simulink model "Model"  (R2024b)
settings: Solver=ode45  StartTime=0.0  StopTime=20  RelTol=1e-3
InitFcn:
  | Design
values from neighbouring files (symbols this model uses):
  A = [0, 1; 0, -1/Tm]    [Design.m]
  B = [0; Km/Tm/gbox.N]    [Design.m]
  C = [1, 0]    [Design.m]
  D = 0    [Design.m]
  K = K(2:end)    [Design.m]
  Ki = K(1)    [Design.m]
  Nr = Nu + K * Nx    [Design.m]
  Nu = tmp(end)    [Design.m]
  Nx = tmp(1:N, 1)    [Design.m]
  Ref = 70    [Design.m]
undefined symbols (not defined in the file or in its folder): daq, drv, ElecDyn, gbox, MechDyn, mot, rads2rpm, RD, sens, Tau_sf, Ts
libraries: simulink_extras x5
settings Model: Creator=Banaan  LastModifiedBy=Banaan

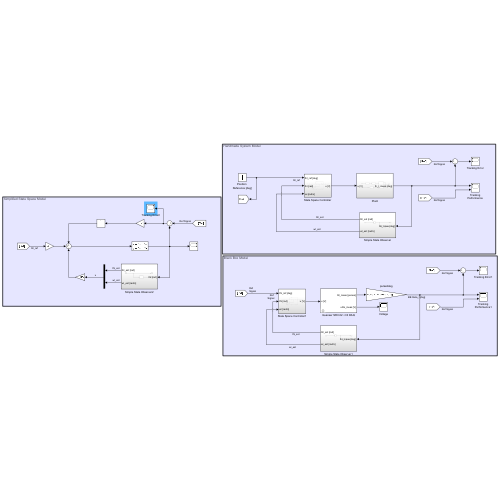
[thumbnail: Simulink's stored preview of the top-level diagram]
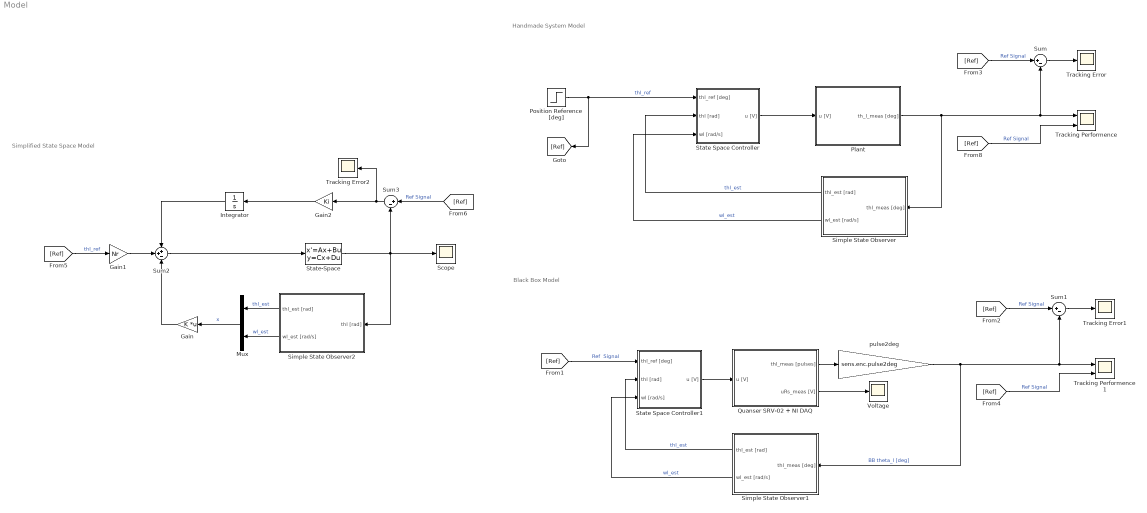
== system Model ==
  note: Simplified State Space Model
  note: Handmade System Model
  note: Black Box Model
  Gain : Gain  Gain=K  Multiplication=Matrix(K*u)
  Gain1 : Gain  Gain=Nr
  Gain2 : Gain  Gain=Ki
  Integrator : Integrator
  Mux : Mux  Inputs=2
  Plant : Subsystem
  Position Reference [deg] : Step  After=Ref  SampleTime=0
  Quanser SRV-02 + NI DAQ : Subsystem  mask(Quanser SRV-02 (with inertial load) + NI DAQ){Ts=0.001, fricType=Coulomb + viscous}
      mask prompts: Ts "NI DAQ Sample Time:"; fricType "Friction model"
      mask help: Quanser SRV-02 (with inertial load) + NI DAQ model.
      mask init:
      | %%  Sensors data
      | 
      | %   shunt resistor
      | sens.curr.Rs = 0.5;                         %   resistance [Ohm]   
      | sens.curr.uRs_std = 0.01;                   %   voltage noise standard dev [V]                           
      | sens.curr.uRs_var = sens.curr.uRs_std^2;	%   voltage noise variance [V^2]
      | 
      | %   Hewlett-Packard HEDS-5540#A06 optical encoder
      | sens.enc.ppr = 500*4;                       %   pulses per rotation
      | sens.enc.pulse2deg = 360/sens.enc.ppr;      %   [pulses] -> [deg]
      | sens.enc.pulse2rad = 2*pi/sens.enc.ppr;     %   [pulses] -> [rad]
      | sens.enc.deg2pulse = sens.enc.ppr/360;      %   [deg] -> [pulses]
      | sens.enc.rad2pulse = sens.enc.ppr/2/pi;     %   [rad] -> [pulses]
      | 
      | 
      | %%  Data acquisition board (daq) data
      | 
      | %   NI PCI-6221 DAC data
      | daq.dac.bits = 16;                                  %   resolution (bits)
      | daq.dac.fs   = 10;                                  %   full scale 
      | daq.dac.q    = 2*daq.dac.fs/(2^daq.dac.bits-1);     %	quantization
      | 
      | %   NI PCI-6221 ADC data
      | daq.adc.bits = 16;                                  %   resolution (bits)
      | daq.adc.fs   = 10;                                  %   full scale (as set in SLDRT Analog Input block)
      | daq.adc.q    = 2*daq.adc.fs/(2^daq.adc.bits-1);     %   quantization
      mask Help:
      | Riccardo Antonello (antonello@dei.unipd.it)
      | 
      | April 24, 2020
      | 
      | Dept. of Information Engineering, University of Padova
      mask TypeOptions fricType: Coulomb + viscous | Karnopp
  Scope : Scope
  Simple State Observer : Subsystem
  Simple State Observer1 : Subsystem
  Simple State Observer2 : Subsystem
  State Space Controller : Subsystem
  State Space Controller1 : Subsystem
  State-Space : StateSpace  A=A  B=B  C=C  D=D  InitialCondition=0
  Sum : Sum  Inputs=|+-
  Sum1 : Sum  Inputs=|+-
  Sum2 : Sum  Inputs=++-
  Sum3 : Sum  Inputs=|+-
  Tracking Performence : Scope  NumInputPorts=2
  Tracking Performence1 : Scope  NumInputPorts=2
  Tracking Error : Scope
  Tracking Error1 : Scope
  Tracking Error2 : Scope
  Voltage : Scope
  pulse2deg : Gain  Gain=sens.enc.pulse2deg
  wires:
  Plant/1(th_l_meas [deg]) -> Sum/2, Tracking Performence/1, Simple State Observer/1(thl_meas [deg])
  Position Reference [deg]/1 -> [Ref], State Space Controller/1(thl_ref [deg])  "thl_ref"
  Quanser SRV-02 + NI DAQ/1(thl_meas [pulses]) -> pulse2deg/1
  pulse2deg/1 -> Simple State Observer1/1(thl_meas [deg]), Tracking Performence1/1, Sum1/2  "BB theta_l [deg]"
  Quanser SRV-02 + NI DAQ/2(uRs_meas [V]) -> Voltage/1
  [Ref] -> State Space Controller1/1(thl_ref [deg])  "Ref  Signal"
  [Ref] -> Tracking Performence/2  "Ref Signal"
  State Space Controller/1(u [V]) -> Plant/1(u [V])
  Simple State Observer/1(thl_est [rad]) -> State Space Controller/2(thl [rad])  "thl_est"
  Simple State Observer/2(wl_est [rad/s]) -> State Space Controller/3(wl [rad/s])  "wl_est"
  [Ref] -> Sum/1  "Ref Signal"
  Sum/1 -> Tracking Error/1
  Sum1/1 -> Tracking Error1/1
  [Ref] -> Sum1/1  "Ref Signal"
  [Ref] -> Tracking Performence1/2  "Ref Signal"
  Simple State Observer1/2(wl_est [rad/s]) -> State Space Controller1/3(wl [rad/s])  "wl_est"
  Simple State Observer1/1(thl_est [rad]) -> State Space Controller1/2(thl [rad])  "thl_est"
  State Space Controller1/1(u [V]) -> Quanser SRV-02 + NI DAQ/1(u [V])
  Simple State Observer2/2(wl_est [rad/s]) -> Mux/2  "wl_est"
  Simple State Observer2/1(thl_est [rad]) -> Mux/1  "thl_est"
  Mux/1 -> Gain/1  "x"
  Gain/1 -> Sum2/3
  Sum2/1 -> State-Space/1
  Gain1/1 -> Sum2/2
  [Ref] -> Gain1/1  "thl_ref"
  [Ref] -> Sum3/1  "Ref Signal"
  Sum3/1 -> Gain2/1, Tracking Error2/1
  State-Space/1 -> Sum3/2, Scope/1, Simple State Observer2/1(thl [rad])
  Gain2/1 -> Integrator/1
  Integrator/1 -> Sum2/1

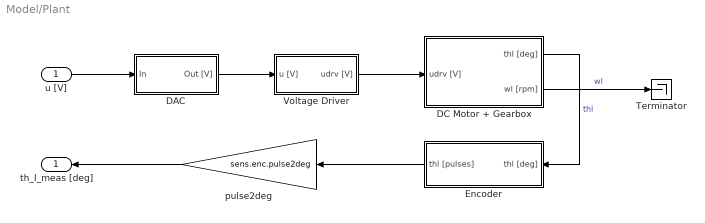
== system Model/Plant ==
  u [V] : Inport
  DAC : Subsystem
  DC Motor + Gearbox : Subsystem
  Encoder : Subsystem
  Terminator : Terminator
  Voltage Driver : Subsystem
  pulse2deg : Gain  Gain=sens.enc.pulse2deg
  th_l_meas [deg] : Outport
  wires:
  DAC/1(Out [V]) -> Voltage Driver/1(u [V])
  Encoder/1(thl [pulses]) -> pulse2deg/1
  u [V]/1 -> DAC/1(In)
  Voltage Driver/1(udrv [V]) -> DC Motor + Gearbox/1(udrv [V])
  DC Motor + Gearbox/2(wl [rpm]) -> Terminator/1  "wl"
  DC Motor + Gearbox/1(thl [deg]) -> Encoder/1(thl [deg])  "thl"
  pulse2deg/1 -> th_l_meas [deg]/1

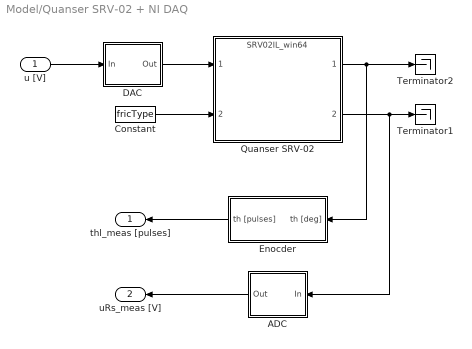
== system Model/Quanser SRV-02 + NI DAQ ==
  u [V] : Inport
  ADC : Subsystem
  Constant : Constant  Value=fricType
  DAC : Subsystem
  Enocder : Subsystem
  Quanser SRV-02 : ModelReference  ModelNameDialog=SRV02IL_win64.slxp  ModelReferenceVersion=1.44  CopyOfModelProtected=on
  Terminator1 : Terminator
  Terminator2 : Terminator
  thl_meas [pulses] : Outport
  uRs_meas [V] : Outport  Port=2
  wires:
  Enocder/1(th [pulses]) -> thl_meas [pulses]/1
  ADC/1(Out) -> uRs_meas [V]/1
  DAC/1(Out) -> Quanser SRV-02/1
  Quanser SRV-02/2 -> ADC/1(In), Terminator1/1
  u [V]/1 -> DAC/1(In)
  Quanser SRV-02/1 -> Enocder/1(th [deg]), Terminator2/1
  Constant/1 -> Quanser SRV-02/2

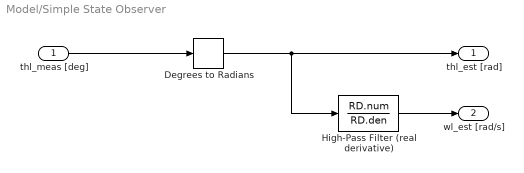
== system Model/Simple State Observer ==
  thl_meas [deg] : Inport
  Degrees to Radians : simulink_extras/Transformations/Degrees to Radians
  High-Pass Filter (real derivative) : TransferFcn  Numerator=RD.num  Denominator=RD.den
  thl_est [rad] : Outport
  wl_est [rad/s] : Outport  Port=2
  wires:
  thl_meas [deg]/1 -> Degrees to Radians/1
  High-Pass Filter (real derivative)/1 -> wl_est [rad/s]/1
  Degrees to Radians/1 -> High-Pass Filter (real derivative)/1, thl_est [rad]/1

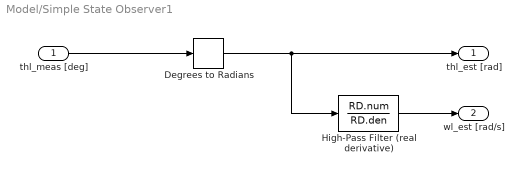
== system Model/Simple State Observer1 ==
  thl_meas [deg] : Inport
  Degrees to Radians : simulink_extras/Transformations/Degrees to Radians
  High-Pass Filter (real derivative) : TransferFcn  Numerator=RD.num  Denominator=RD.den
  thl_est [rad] : Outport
  wl_est [rad/s] : Outport  Port=2
  wires:
  High-Pass Filter (real derivative)/1 -> wl_est [rad/s]/1
  Degrees to Radians/1 -> High-Pass Filter (real derivative)/1, thl_est [rad]/1
  thl_meas [deg]/1 -> Degrees to Radians/1

== system Model/Simple State Observer2 ==
  thl [rad] : Inport
  High-Pass Filter (real derivative) : TransferFcn  Numerator=RD.num  Denominator=RD.den
  thl_est [rad] : Outport
  wl_est [rad/s] : Outport  Port=2
  wires:
  High-Pass Filter (real derivative)/1 -> wl_est [rad/s]/1
  thl [rad]/1 -> thl_est [rad]/1, High-Pass Filter (real derivative)/1

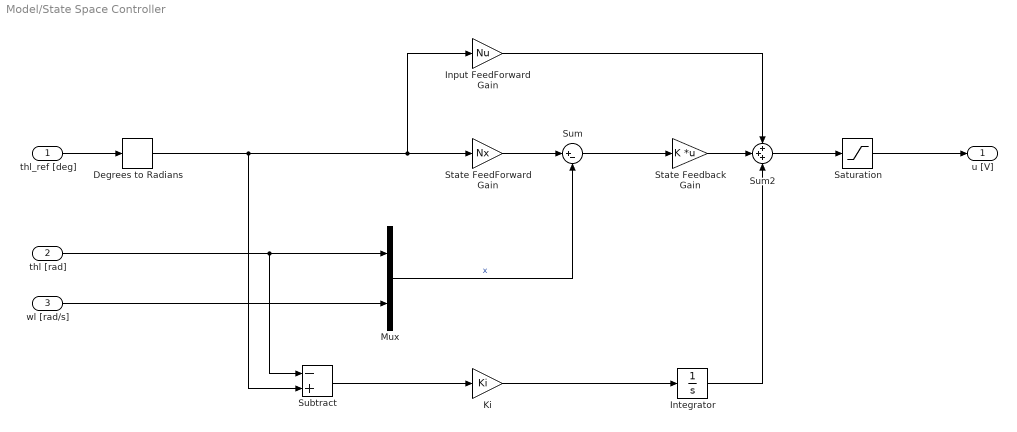
== system Model/State Space Controller ==
  thl_ref [deg] : Inport
  thl [rad] : Inport  Port=2
  wl [rad/s] : Inport  Port=3
  Degrees to Radians : simulink_extras/Transformations/Degrees to Radians
  Input FeedForward Gain : Gain  Gain=Nu
  Integrator : Integrator
  Ki : Gain  Gain=Ki
  Mux : Mux  Inputs=2
  Saturation : Saturate  UpperLimit=daq.adc.fs  LowerLimit=-daq.adc.fs
  State FeedForward Gain : Gain  Gain=Nx
  State Feedback Gain : Gain  Gain=K  Multiplication=Matrix(K*u)
  Subtract : Sum  Inputs=-+
  Sum : Sum  Inputs=|+-
  Sum2 : Sum  Inputs=+++
  u [V] : Outport
  wires:
  Sum/1 -> State Feedback Gain/1
  Mux/1 -> Sum/2  "x"
  thl_ref [deg]/1 -> Degrees to Radians/1
  State FeedForward Gain/1 -> Sum/1
  State Feedback Gain/1 -> Sum2/2
  Input FeedForward Gain/1 -> Sum2/1
  Sum2/1 -> Saturation/1
  Saturation/1 -> u [V]/1
  Degrees to Radians/1 -> Subtract/2, Input FeedForward Gain/1, State FeedForward Gain/1
  thl [rad]/1 -> Subtract/1, Mux/1
  wl [rad/s]/1 -> Mux/2
  Subtract/1 -> Ki/1
  Ki/1 -> Integrator/1
  Integrator/1 -> Sum2/3

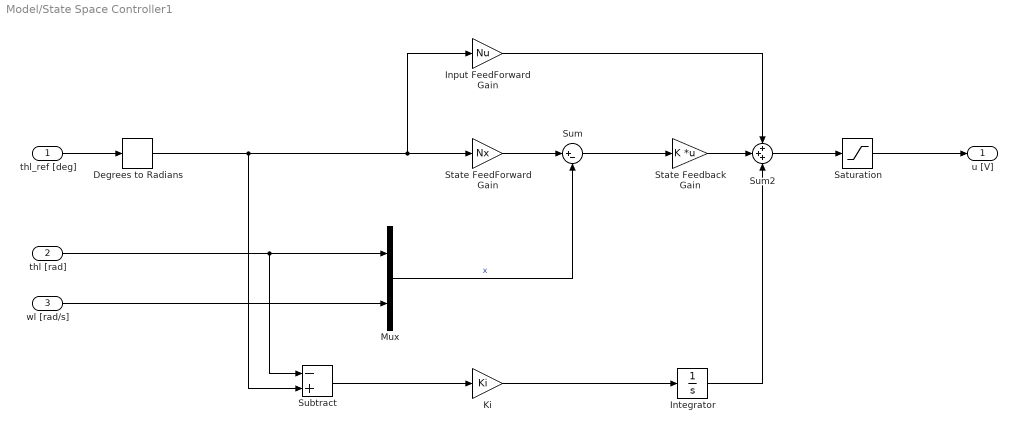
== system Model/State Space Controller1 ==
  thl_ref [deg] : Inport
  thl [rad] : Inport  Port=2
  wl [rad/s] : Inport  Port=3
  Degrees to Radians : simulink_extras/Transformations/Degrees to Radians
  Input FeedForward Gain : Gain  Gain=Nu
  Integrator : Integrator
  Ki : Gain  Gain=Ki
  Mux : Mux  Inputs=2
  Saturation : Saturate  UpperLimit=daq.adc.fs  LowerLimit=-daq.adc.fs
  State FeedForward Gain : Gain  Gain=Nx
  State Feedback Gain : Gain  Gain=K  Multiplication=Matrix(K*u)
  Subtract : Sum  Inputs=-+
  Sum : Sum  Inputs=|+-
  Sum2 : Sum  Inputs=+++
  u [V] : Outport
  wires:
  Saturation/1 -> u [V]/1
  Sum/1 -> State Feedback Gain/1
  wl [rad/s]/1 -> Mux/2
  Ki/1 -> Integrator/1
  Subtract/1 -> Ki/1
  State FeedForward Gain/1 -> Sum/1
  Sum2/1 -> Saturation/1
  thl_ref [deg]/1 -> Degrees to Radians/1
  Degrees to Radians/1 -> Subtract/2, Input FeedForward Gain/1, State FeedForward Gain/1
  thl [rad]/1 -> Subtract/1, Mux/1
  Input FeedForward Gain/1 -> Sum2/1
  Mux/1 -> Sum/2  "x"
  State Feedback Gain/1 -> Sum2/2
  Integrator/1 -> Sum2/3

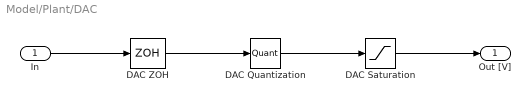
== system Model/Plant/DAC ==
  In : Inport
  DAC Quantization : Quantizer  QuantizationInterval=daq.dac.q
  DAC Saturation : Saturate  UpperLimit=daq.dac.fs  LowerLimit=-daq.dac.fs
  DAC ZOH : ZeroOrderHold  SampleTime=Ts
  Out [V] : Outport
  wires:
  DAC Quantization/1 -> DAC Saturation/1
  DAC ZOH/1 -> DAC Quantization/1
  DAC Saturation/1 -> Out [V]/1
  In/1 -> DAC ZOH/1

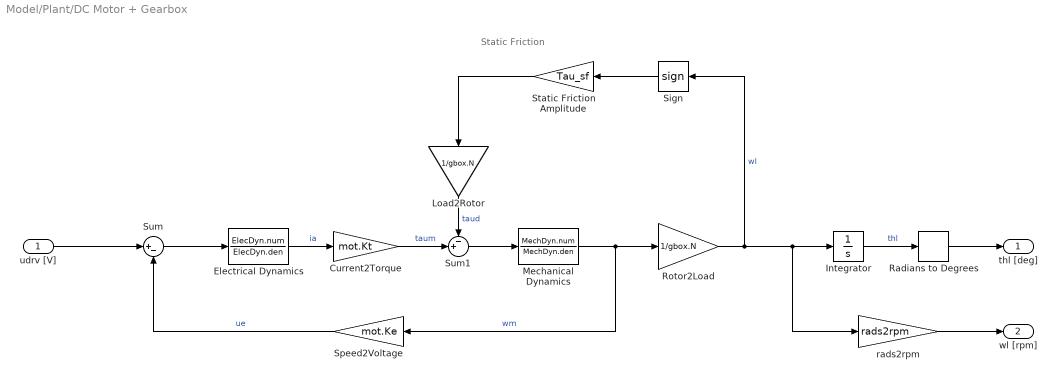
== system Model/Plant/DC Motor + Gearbox ==
  note: Static Friction
  udrv [V] : Inport
  Current2Torque : Gain  Gain=mot.Kt
  Electrical Dynamics : TransferFcn  Numerator=ElecDyn.num  Denominator=ElecDyn.den
  Integrator : Integrator
  Load2Rotor : Gain  Gain=1/gbox.N
  Mechanical Dynamics : TransferFcn  Numerator=MechDyn.num  Denominator=MechDyn.den
  Radians to Degrees : simulink_extras/Transformations/Radians to Degrees
  Rotor2Load : Gain  Gain=1/gbox.N
  Sign : Signum  ZeroCross=off
  Speed2Voltage : Gain  Gain=mot.Ke
  Static Friction Amplitude : Gain  Gain=Tau_sf
  Sum : Sum  Inputs=|+-
  Sum1 : Sum  Inputs=-+|
  rads2rpm : Gain  Gain=rads2rpm
  thl [deg] : Outport
  wl [rpm] : Outport  Port=2
  wires:
  Rotor2Load/1 -> rads2rpm/1, Integrator/1, Sign/1  "wl"
  Electrical Dynamics/1 -> Current2Torque/1  "ia"
  Sum1/1 -> Mechanical Dynamics/1
  Speed2Voltage/1 -> Sum/2  "ue"
  Load2Rotor/1 -> Sum1/1  "taud"
  Radians to Degrees/1 -> thl [deg]/1
  Mechanical Dynamics/1 -> Speed2Voltage/1, Rotor2Load/1  "wm"
  Sum/1 -> Electrical Dynamics/1
  Integrator/1 -> Radians to Degrees/1  "thl"
  Current2Torque/1 -> Sum1/2  "taum"
  rads2rpm/1 -> wl [rpm]/1
  Sign/1 -> Static Friction Amplitude/1
  Static Friction Amplitude/1 -> Load2Rotor/1
  udrv [V]/1 -> Sum/1

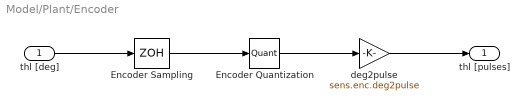
== system Model/Plant/Encoder ==
  thl [deg] : Inport
  Encoder Quantization : Quantizer  QuantizationInterval=daq.adc.q
  Encoder Sampling : ZeroOrderHold  SampleTime=Ts
  deg2pulse : Gain  Gain=sens.enc.deg2pulse
  thl [pulses] : Outport
  wires:
  Encoder Sampling/1 -> Encoder Quantization/1
  Encoder Quantization/1 -> deg2pulse/1
  thl [deg]/1 -> Encoder Sampling/1
  deg2pulse/1 -> thl [pulses]/1

== system Model/Plant/Voltage Driver ==
  u [V] : Inport
  Driver Dynamics : TransferFcn  Numerator=drv.dcgain  Denominator=[drv.Tc, 1]
  Driver Saturation : Saturate  UpperLimit=drv.outmax  LowerLimit=-drv.outmax
  udrv [V] : Outport
  wires:
  Driver Dynamics/1 -> Driver Saturation/1
  u [V]/1 -> Driver Dynamics/1
  Driver Saturation/1 -> udrv [V]/1

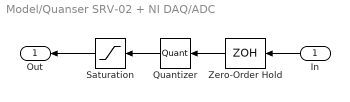
== system Model/Quanser SRV-02 + NI DAQ/ADC ==
  In : Inport
  Quantizer : Quantizer  QuantizationInterval=daq.adc.q
  Saturation : Saturate  UpperLimit=daq.adc.fs  LowerLimit=-daq.adc.fs
  Zero-Order Hold : ZeroOrderHold  SampleTime=Ts
  Out : Outport
  wires:
  Saturation/1 -> Out/1
  In/1 -> Zero-Order Hold/1
  Quantizer/1 -> Saturation/1
  Zero-Order Hold/1 -> Quantizer/1

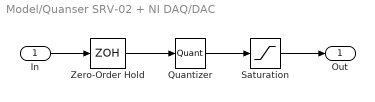
== system Model/Quanser SRV-02 + NI DAQ/DAC ==
  In : Inport
  Quantizer : Quantizer  QuantizationInterval=daq.dac.q
  Saturation : Saturate  UpperLimit=daq.dac.fs  LowerLimit=-daq.dac.fs
  Zero-Order Hold : ZeroOrderHold  SampleTime=Ts
  Out : Outport
  wires:
  Quantizer/1 -> Saturation/1
  In/1 -> Zero-Order Hold/1
  Zero-Order Hold/1 -> Quantizer/1
  Saturation/1 -> Out/1

== system Model/Quanser SRV-02 + NI DAQ/Enocder ==
  th [deg] : Inport
  Quantizer : Quantizer  QuantizationInterval=sens.enc.pulse2deg
  Zero-Order Hold : ZeroOrderHold  SampleTime=Ts
  deg2pulse : Gain  Gain=sens.enc.deg2pulse
  th [pulses] : Outport
  wires:
  Quantizer/1 -> deg2pulse/1
  th [deg]/1 -> Zero-Order Hold/1
  Zero-Order Hold/1 -> Quantizer/1
  deg2pulse/1 -> th [pulses]/1
